simulink model "P5_8_Quad_PID"  (R2025b)
settings: Solver=ode45  StartTime=0.0  StopTime=10.0  MaxStep=1e-2  RelTol=1e-3  AbsTol=1e-4
settings Model: Creator=tongx  LastModifiedBy=tongx

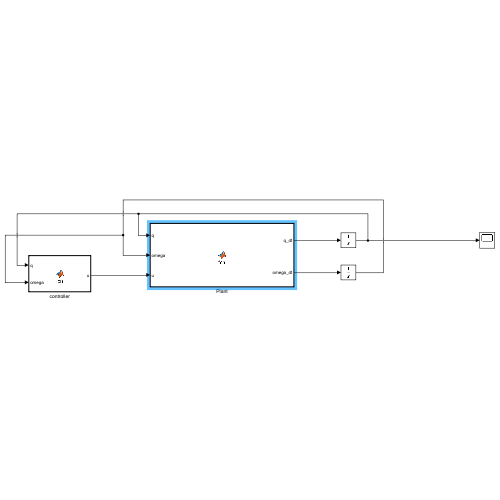
[thumbnail: Simulink's stored preview of the top-level diagram]
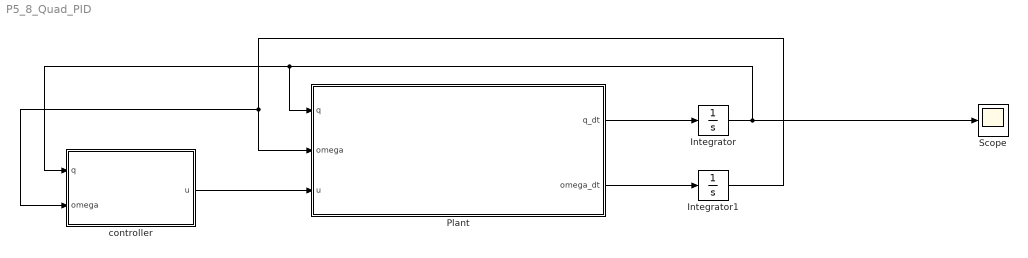
== system P5_8_Quad_PID ==
  Integrator : Integrator  InitialCondition=[0 1 0 0].'
  Integrator1 : Integrator  InitialCondition=[0 0 3].'
  Plant : MATLAB Function  TreatAsAtomicUnit=on
  Scope : Scope
      settings: ActiveDisplayYMinimum=-1  ActiveDisplayYMaximum=1
  controller : MATLAB Function  TreatAsAtomicUnit=on
  wires:
  Plant/1(q_dt) -> Integrator/1
  Integrator/1 -> Scope/1, controller/1(q), Plant/1(q)
  Plant/2(omega_dt) -> Integrator1/1
  Integrator1/1 -> controller/2(omega), Plant/2(omega)
  controller/1(u) -> Plant/3(u)

== matlab function P5_8_Quad_PID/controller ==
  data: q input; u output; omega input
function u = fcn(q, omega)

kp = 20;

kd = 10;

u = -kp*q(2:4)-kd*omega;

== matlab function P5_8_Quad_PID/Plant ==
  data: q input; omega input; u input; q_dt output; omega_dt output
function [q_dt, omega_dt] = fcn(q, omega, u)

J = diag([1,2,3]);

Sw = [0 -omega(3) omega(2)
    omega(3) 0 -omega(1)
    -omega(2) omega(1) 0];

q_dt = [0 -omega.'
    omega -Sw]*q;


omega_dt = inv(J)*(-Sw*J*omega + u);
